simulink model "Temp_controlSysid"  (R2016b)
settings: Solver=FixedStepAuto  StartTime=0.0  StopTime=20000  RelTol=1e-3  EnableMultiTasking=on
undefined symbols (not defined in the file or in its folder): DiscIntNeverNeededParam
libraries: simulink x35, simulink_need_slupdate x5, EEE481Arduino x1
settings Model: ExtModeTrigDuration=2  Creator=EliteBook 8470p  LastModifiedBy=rsjoshi1
settings OptimizationCC: LifeSpan=1  MaxStackSize=64
settings DebuggingCC: SFUnexpectedBacktrackingDiag=warning  SFNoUnconditionalDefaultTransitionDiag=warning  SFExecutionAtInitializationDiag=none
settings HardwareCC: ProdBitPerPointer=32  ProdBitPerSizeT=32  ProdBitPerPtrDiffT=32  ProdLargestAtomicInteger=Long  ProdLargestAtomicFloat=Double  ProdWordSize=32  ProdHWDeviceType=ARM Compatible->ARM Cortex
settings RTWCC: SystemTargetFile=ert.tlc  HardwareBoard=Arduino Due  TLCOptions=-aInlineSetEventsForThisBaseRateFcn=TLC_FALSE -aSuppressMultiTaskScheduler=TLC_FALSE -aRateBasedStepFcn=1  TemplateMakefile=ert_default_tmf  Description=Embedded Coder  GenerateReport=on  Toolchain=Arduino ARM v1.6.7  BuildConfiguration=Faster Runs  IncludeHyperlinkInReport=on  LaunchReport=on  GenerateTraceInfo=on  GenerateTraceReport=on  GenerateTraceReportSl=on  GenerateTraceReportSf=on  GenerateTraceReportEml=on
settings CodeAppCC: ForceParamTrailComments=on  IgnoreCustomStorageClasses=off  OperatorAnnotations=on  SimulinkDataObjDesc=on  SFDataObjDesc=on  MATLABFcnDesc=on  InsertBlockDesc=on  MATLABSourceComments=on
settings ERTTargetCC: SupportContinuousTime=on  SupportVariableSizeSignals=on
settings ConfigComp: CovMetricSettings=dw  CovHtmlReporting=on  CovSaveCumulativeToWorkspaceVar=on  CovSaveSingleToWorkspaceVar=on  CovExternalEMLEnable=off

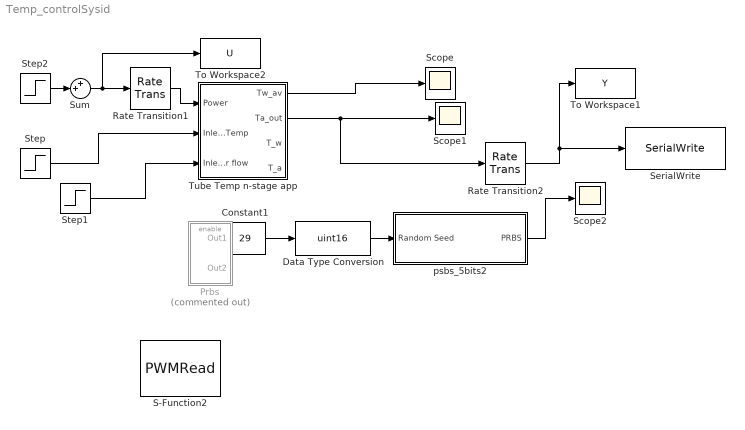
== system Temp_controlSysid ==
  Constant1 : Constant  Value=29  OutDataTypeStr=double  SampleTime=1
  Data Type Conversion : DataTypeConversion  OutDataTypeStr=uint16
  Prbs : Subsystem  Commented=on
  Rate Transition1 : RateTransition  OutPortSampleTimeOpt=Inherit  OutPortSampleTime=0.05
  Rate Transition2 : RateTransition  OutPortSampleTimeOpt=Inherit  OutPortSampleTime=0.05
  S-Function2 : S-Function  FunctionName=PWMRead  SFunctionModules=PWMRead_wrapper  SFunctionDeploymentMode=off  EnableBusSupport=off
  Scope : Scope
  Scope1 : Scope
  Scope2 : Scope
  SerialWrite : EEE481Arduino/SerialWrite  serialNum=2
  Step : Step  Time=10000  Before=25  After=25  SampleTime=0
  Step1 : Step  Time=5000  Before=1  SampleTime=0
  Step2 : Step  Time=100  After=0.49  SampleTime=1
  Sum : Sum  Inputs=++|
  To Workspace1 : ToWorkspace  VariableName=Y  SampleTime=1
  To Workspace2 : ToWorkspace  VariableName=U  SampleTime=1
  Tube Temp n-stage app : Subsystem  mask{L=0.5, n=10, ra=0.1, T_01=800, T_a01=25, T_amb=25}
      mask prompts: L "Tube Length"; n "Number of sections"; ra "Tube inner radius"; T_01 "Initial tube temp"; T_a01 "Initial air temp"; T_amb "Ambient Temp"
      mask init:
      | cp=1078;cpa=1134;rhoa=0.5;hs=5;ha=30;rhos=2500;k=2;
      | d=.01;vt=pi*L*((ra+d)*(ra+d)-ra*ra);m=vt*rhos;
      | As=2*pi*(ra+.1)*L;V=pi*ra*ra*L;Aa=2*pi*ra*L;
      | A_d=pi*((ra+d)*(ra+d)-ra*ra);A_rat=1;Li=L/n;
      | T_0=T_01*ones(n,1);T_a0=T_a01*ones(n,1);
  psbs_5bits2 : Subsystem  mask(PRBS with 8 shift registers){T=1, Tsw=200, Lz=12000, Lv=0.1, Nc=1}
      mask prompts: T "Sample Time (s)"; Tsw "Time to switch (s)"; Lz "Leading Zeros (s)"; Lv "Switching Levels"; Nc "Number of Cycles"
      mask help:
      | Creates a PRBS signal using 6 shift registers.
      |     *Time to switch (Tsw) must be an integer multiple of Sample Time (T).
      |     *Leading zeros specify how long the PRBS will be zero, in seconds, before the levels begin shifting.
      |     *Level is the amplitude of the desired PRBS signal. Both + and - levels are equal
      |     *Number of cycles determines the number of full cycles generated. Each cycle is (2^6-1)*Tsw seconds long
  wires:
  Step1/1 -> Tube Temp n-stage app/3(Inlet Air flow)
  Step/1 -> Tube Temp n-stage app/2(Inlet Air Temp)
  Tube Temp n-stage app/2(Ta_out) -> Rate Transition2/1, Scope1/1
  Tube Temp n-stage app/1(Tw_av) -> Scope/1
  psbs_5bits2/1(PRBS) -> Scope2/1
  Constant1/1 -> Data Type Conversion/1
  Data Type Conversion/1 -> psbs_5bits2/1(Random Seed)
  Step2/1 -> Sum/2
  Sum/1 -> To Workspace2/1, Rate Transition1/1
  Rate Transition1/1 -> Tube Temp n-stage app/1(Power)
  Rate Transition2/1 -> To Workspace1/1, SerialWrite/1

== system Temp_controlSysid/Prbs ==
  Enable : EnablePort
  Constant1 : Constant  Value=29  OutDataTypeStr=double  SampleTime=0.1
  Constant2 : Constant  Value=30  OutDataTypeStr=double  SampleTime=0.1
  Data Type Conversion : DataTypeConversion  OutDataTypeStr=uint16
  Data Type Conversion2 : DataTypeConversion  OutDataTypeStr=uint16
  Rate Transition1 : RateTransition  OutPortSampleTime=0.1
  Rate Transition2 : RateTransition  OutPortSampleTime=0.1
  psbs_5bits1 : Subsystem  mask(PRBS with 8 shift registers){T=0.1, Tsw=20, Lz=10, Lv=300, Nc=1}
      mask prompts: T "Sample Time (s)"; Tsw "Time to switch (s)"; Lz "Leading Zeros (s)"; Lv "Switching Levels"; Nc "Number of Cycles"
      mask help:
      | Creates a PRBS signal using 6 shift registers.
      |     *Time to switch (Tsw) must be an integer multiple of Sample Time (T).
      |     *Leading zeros specify how long the PRBS will be zero, in seconds, before the levels begin shifting.
      |     *Level is the amplitude of the desired PRBS signal. Both + and - levels are equal
      |     *Number of cycles determines the number of full cycles generated. Each cycle is (2^6-1)*Tsw seconds long
  psbs_5bits2 : Subsystem  mask(PRBS with 8 shift registers){T=0.1, Tsw=20, Lz=10, Lv=300, Nc=1}
      mask prompts: T "Sample Time (s)"; Tsw "Time to switch (s)"; Lz "Leading Zeros (s)"; Lv "Switching Levels"; Nc "Number of Cycles"
      mask help:
      | Creates a PRBS signal using 6 shift registers.
      |     *Time to switch (Tsw) must be an integer multiple of Sample Time (T).
      |     *Leading zeros specify how long the PRBS will be zero, in seconds, before the levels begin shifting.
      |     *Level is the amplitude of the desired PRBS signal. Both + and - levels are equal
      |     *Number of cycles determines the number of full cycles generated. Each cycle is (2^6-1)*Tsw seconds long
  psbs_7bits1 : Subsystem  Commented=on  mask(PRBS with 8 shift registers){T=0.1, Tsw=60, Lz=10, Lv=300, Nc=1}
      mask prompts: T "Sample Time (s)"; Tsw "Time to switch (s)"; Lz "Leading Zeros (s)"; Lv "Switching Levels"; Nc "Number of Cycles"
      mask help:
      | Creates a PRBS signal using 7 shift registers.
      |     *Time to switch (Tsw) must be an integer multiple of Sample Time (T).
      |     *Leading zeros specify how long the PRBS will be zero, in seconds, before the levels begin shifting.
      |     *Level is the amplitude of the desired PRBS signal. Both + and - levels are equal
      |     *Number of cycles determines the number of full cycles generated. Each cycle is (2^7-1)*Tsw seconds long
  psbs_8bits2 : Subsystem  Commented=on  mask(PRBS with 8 shift registers){T=0.1, Tsw=20, Lz=50, Lv=300, Nc=1}
      mask prompts: T "Sample Time (s)"; Tsw "Time to switch (s)"; Lz "Leading Zeros (s)"; Lv "Switching Levels"; Nc "Number of Cycles"
      mask help:
      | Creates a PRBS signal using 8 shift registers.
      |     *Time to switch (Tsw) must be an integer multiple of Sample Time (T).
      |     *Leading zeros specify how long the PRBS will be zero, in seconds, before the levels begin shifting.
      |     *Level is the amplitude of the desired PRBS signal. Both + and - levels are equal
      |     *Number of cycles determines the number of full cycles generated. Each cycle is (2^8-1)*Tsw seconds long
  Out1 : Outport
  Out2 : Outport  Port=2
  wires:
  Constant1/1 -> Data Type Conversion/1
  Data Type Conversion/1 -> Rate Transition1/1
  psbs_5bits2/1(PRBS) -> Out1/1
  Rate Transition1/1 -> psbs_5bits2/1(Random Seed)
  psbs_5bits1/1(PRBS) -> Out2/1
  Rate Transition2/1 -> psbs_5bits1/1(Random Seed)
  Constant2/1 -> Data Type Conversion2/1
  Data Type Conversion2/1 -> Rate Transition2/1

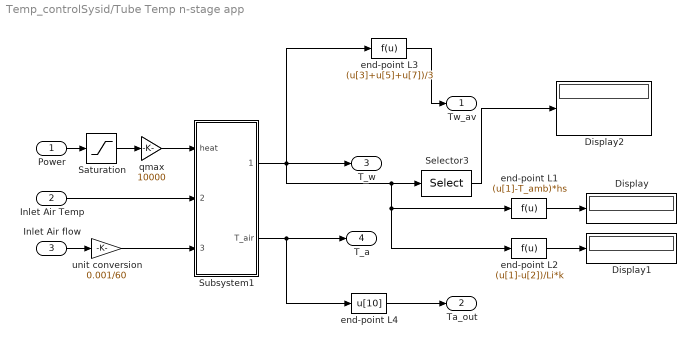
== system Temp_controlSysid/Tube Temp n-stage app ==
  Power : Inport
  Inlet Air Temp : Inport  Port=2
  Inlet Air flow : Inport  Port=3
  Display : Display
      settings: Format=short_e
  Display1 : Display
      settings: Format=short_e
  Display2 : Display
      settings: Format=short_e
  Saturation : Saturate  UpperLimit=1  LowerLimit=0
  Selector3 : Selector  InputPortWidth=n  IndexOptions=Index vector (dialog)  Indices=[1,2]  OutputSizes=1
  Subsystem1 : Subsystem
  end-point L1 : Fcn  Expr=(u[1]-T_amb)*hs
  end-point L2 : Fcn  Expr=(u[1]-u[2])/Li*k
  end-point L3 : Fcn  Expr=(u[3]+u[5]+u[7])/3
  end-point L4 : Fcn  Expr=u[10]
  qmax : Gain  Gain=10000  SaturateOnIntegerOverflow=on  OutDataTypeStr=Inherit: Same as input  ParamDataTypeStr=Inherit: Same as input
  unit conversion : Gain  Gain=0.001/60  SaturateOnIntegerOverflow=on  OutDataTypeStr=Inherit: Same as input  ParamDataTypeStr=Inherit: Same as input
  Tw_av : Outport
  Ta_out : Outport  Port=2
  T_w : Outport  Port=3
  T_a : Outport  Port=4
  wires:
  end-point L2/1 -> Display1/1
  end-point L1/1 -> Display/1
  Selector3/1 -> Display2/1
  Subsystem1/2(T_air) -> end-point L4/1, T_a/1
  Subsystem1/1(T_wall) -> end-point L3/1, end-point L2/1, end-point L1/1, Selector3/1, T_w/1
  unit conversion/1 -> Subsystem1/3(Air flow)
  Inlet Air flow/1 -> unit conversion/1
  Power/1 -> Saturation/1
  Saturation/1 -> qmax/1
  Inlet Air Temp/1 -> Subsystem1/2(T_a_inlet)
  qmax/1 -> Subsystem1/1(heat)
  end-point L3/1 -> Tw_av/1
  end-point L4/1 -> Ta_out/1

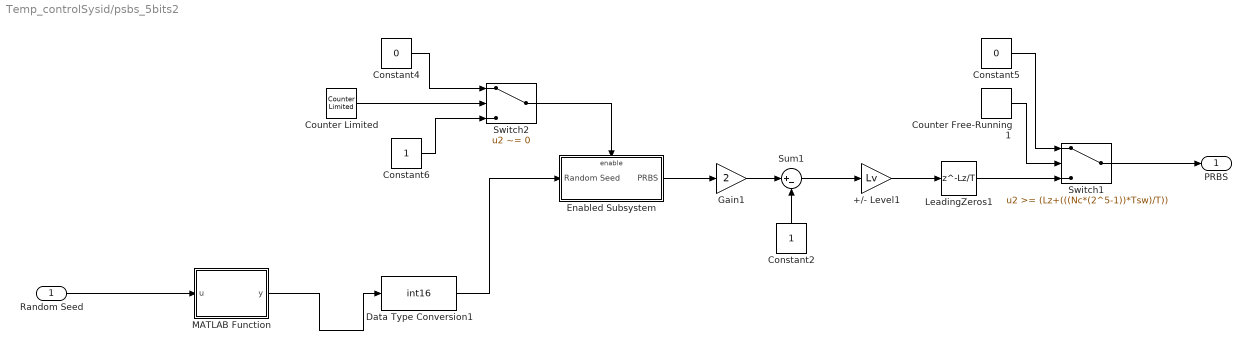
== system Temp_controlSysid/psbs_5bits2 ==
  Random Seed : Inport  OutDataTypeStr=uint16
  +/- Level1 : Gain  Gain=Lv  SampleTime=T
  Constant2 : Constant  SampleTime=T
  Constant4 : Constant  Value=0  SampleTime=T
  Constant5 : Constant  Value=0  SampleTime=T
  Constant6 : Constant  SampleTime=T
  Counter Free-Running1 : simulink/Sources/Counter Free-Running  NumBits=32  tsamp=T
  Counter Limited : simulink/Sources/Counter Limited  uplimit=Tsw/T-1  tsamp=T
  Data Type Conversion1 : DataTypeConversion  OutDataTypeStr=int16
  Enabled Subsystem : Subsystem  TreatAsAtomicUnit=on
  Gain1 : Gain  Gain=2  SampleTime=T
  LeadingZeros1 : Delay  DelayLength=Lz/T  InitialCondition=0  SampleTime=T
  MATLAB Function : MATLAB Function  TreatAsAtomicUnit=on
  Sum1 : Sum  Inputs=|+-  SampleTime=T
  Switch1 : Switch  Threshold=(Lz+(((Nc*(2^5-1))*Tsw)/T))  SampleTime=T
  Switch2 : Switch  Criteria=u2 ~= 0  Threshold=Tsw/T  SampleTime=T
  PRBS : Outport
  wires:
  Switch1/1 -> PRBS/1
  Random Seed/1 -> MATLAB Function/1(u)
  MATLAB Function/1(y) -> Data Type Conversion1/1
  LeadingZeros1/1 -> Switch1/3
  Constant5/1 -> Switch1/1
  +/- Level1/1 -> LeadingZeros1/1
  Counter Free-Running1/1 -> Switch1/2
  Constant2/1 -> Sum1/2
  Gain1/1 -> Sum1/1
  Sum1/1 -> +/- Level1/1
  Enabled Subsystem/1(PRBS) -> Gain1/1
  Data Type Conversion1/1 -> Enabled Subsystem/1(Random Seed)
  Constant6/1 -> Switch2/3
  Constant4/1 -> Switch2/1
  Switch2/1 -> Enabled Subsystem/Enable
  Counter Limited/1 -> Switch2/2

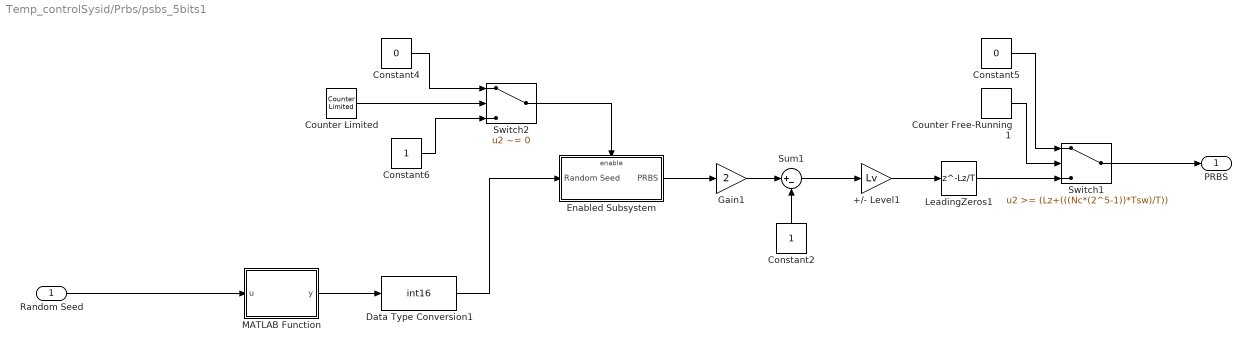
== system Temp_controlSysid/Prbs/psbs_5bits1 ==
  Random Seed : Inport  OutDataTypeStr=uint16
  +/- Level1 : Gain  Gain=Lv  SampleTime=T
  Constant2 : Constant  SampleTime=T
  Constant4 : Constant  Value=0  SampleTime=T
  Constant5 : Constant  Value=0  SampleTime=T
  Constant6 : Constant  SampleTime=T
  Counter Free-Running1 : simulink/Sources/Counter Free-Running  NumBits=32  tsamp=T
  Counter Limited : simulink/Sources/Counter Limited  uplimit=Tsw/T-1  tsamp=T
  Data Type Conversion1 : DataTypeConversion  OutDataTypeStr=int16
  Enabled Subsystem : Subsystem  TreatAsAtomicUnit=on
  Gain1 : Gain  Gain=2  SampleTime=T
  LeadingZeros1 : Delay  DelayLength=Lz/T  InitialCondition=0  SampleTime=T
  MATLAB Function : MATLAB Function  TreatAsAtomicUnit=on
  Sum1 : Sum  Inputs=|+-  SampleTime=T
  Switch1 : Switch  Threshold=(Lz+(((Nc*(2^5-1))*Tsw)/T))  SampleTime=T
  Switch2 : Switch  Criteria=u2 ~= 0  Threshold=Tsw/T  SampleTime=T
  PRBS : Outport
  wires:
  Counter Limited/1 -> Switch2/2
  Switch2/1 -> Enabled Subsystem/Enable
  Constant4/1 -> Switch2/1
  Constant6/1 -> Switch2/3
  Data Type Conversion1/1 -> Enabled Subsystem/1(Random Seed)
  Enabled Subsystem/1(PRBS) -> Gain1/1
  Sum1/1 -> +/- Level1/1
  Gain1/1 -> Sum1/1
  Constant2/1 -> Sum1/2
  Counter Free-Running1/1 -> Switch1/2
  +/- Level1/1 -> LeadingZeros1/1
  Constant5/1 -> Switch1/1
  LeadingZeros1/1 -> Switch1/3
  MATLAB Function/1(y) -> Data Type Conversion1/1
  Random Seed/1 -> MATLAB Function/1(u)
  Switch1/1 -> PRBS/1

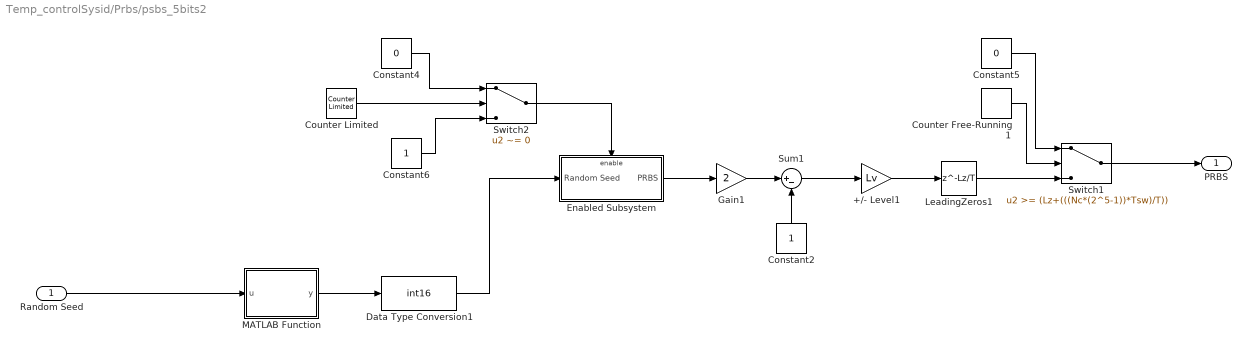
== system Temp_controlSysid/Prbs/psbs_5bits2 ==
  Random Seed : Inport  OutDataTypeStr=uint16
  +/- Level1 : Gain  Gain=Lv  SampleTime=T
  Constant2 : Constant  SampleTime=T
  Constant4 : Constant  Value=0  SampleTime=T
  Constant5 : Constant  Value=0  SampleTime=T
  Constant6 : Constant  SampleTime=T
  Counter Free-Running1 : simulink/Sources/Counter Free-Running  NumBits=32  tsamp=T
  Counter Limited : simulink/Sources/Counter Limited  uplimit=Tsw/T-1  tsamp=T
  Data Type Conversion1 : DataTypeConversion  OutDataTypeStr=int16
  Enabled Subsystem : Subsystem  TreatAsAtomicUnit=on
  Gain1 : Gain  Gain=2  SampleTime=T
  LeadingZeros1 : Delay  DelayLength=Lz/T  InitialCondition=0  SampleTime=T
  MATLAB Function : MATLAB Function  TreatAsAtomicUnit=on
  Sum1 : Sum  Inputs=|+-  SampleTime=T
  Switch1 : Switch  Threshold=(Lz+(((Nc*(2^5-1))*Tsw)/T))  SampleTime=T
  Switch2 : Switch  Criteria=u2 ~= 0  Threshold=Tsw/T  SampleTime=T
  PRBS : Outport
  wires:
  Switch1/1 -> PRBS/1
  Random Seed/1 -> MATLAB Function/1(u)
  MATLAB Function/1(y) -> Data Type Conversion1/1
  LeadingZeros1/1 -> Switch1/3
  Constant5/1 -> Switch1/1
  +/- Level1/1 -> LeadingZeros1/1
  Counter Free-Running1/1 -> Switch1/2
  Constant2/1 -> Sum1/2
  Gain1/1 -> Sum1/1
  Sum1/1 -> +/- Level1/1
  Enabled Subsystem/1(PRBS) -> Gain1/1
  Data Type Conversion1/1 -> Enabled Subsystem/1(Random Seed)
  Constant6/1 -> Switch2/3
  Constant4/1 -> Switch2/1
  Switch2/1 -> Enabled Subsystem/Enable
  Counter Limited/1 -> Switch2/2

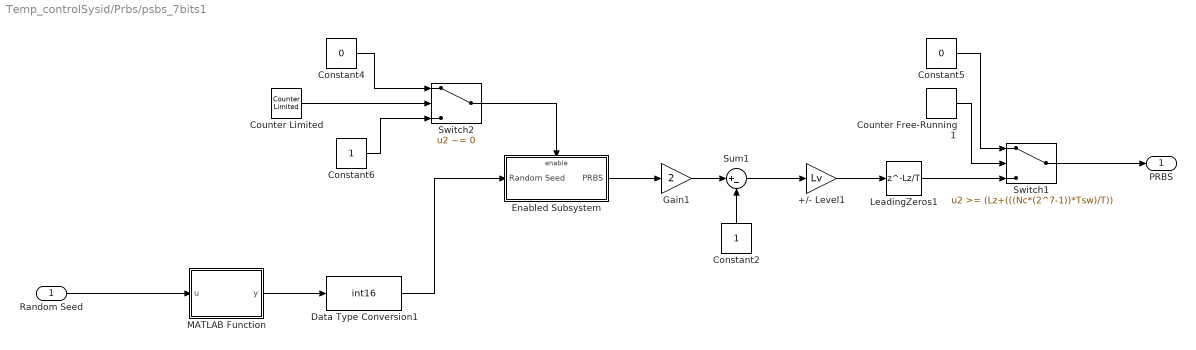
== system Temp_controlSysid/Prbs/psbs_7bits1 ==
  Random Seed : Inport  OutDataTypeStr=uint16
  +/- Level1 : Gain  Gain=Lv  SampleTime=T
  Constant2 : Constant  SampleTime=T
  Constant4 : Constant  Value=0  SampleTime=T
  Constant5 : Constant  Value=0  SampleTime=T
  Constant6 : Constant  SampleTime=T
  Counter Free-Running1 : simulink/Sources/Counter Free-Running  NumBits=32  tsamp=T
  Counter Limited : simulink/Sources/Counter Limited  uplimit=Tsw/T-1  tsamp=T
  Data Type Conversion1 : DataTypeConversion  OutDataTypeStr=int16
  Enabled Subsystem : Subsystem  TreatAsAtomicUnit=on
  Gain1 : Gain  Gain=2  SampleTime=T
  LeadingZeros1 : Delay  DelayLength=Lz/T  InitialCondition=0  SampleTime=T
  MATLAB Function : MATLAB Function  TreatAsAtomicUnit=on
  Sum1 : Sum  Inputs=|+-  SampleTime=T
  Switch1 : Switch  Threshold=(Lz+(((Nc*(2^7-1))*Tsw)/T))  SampleTime=T
  Switch2 : Switch  Criteria=u2 ~= 0  Threshold=Tsw/T  SampleTime=T
  PRBS : Outport
  wires:
  Switch1/1 -> PRBS/1
  Random Seed/1 -> MATLAB Function/1(u)
  MATLAB Function/1(y) -> Data Type Conversion1/1
  LeadingZeros1/1 -> Switch1/3
  Constant5/1 -> Switch1/1
  +/- Level1/1 -> LeadingZeros1/1
  Counter Free-Running1/1 -> Switch1/2
  Constant2/1 -> Sum1/2
  Gain1/1 -> Sum1/1
  Sum1/1 -> +/- Level1/1
  Enabled Subsystem/1(PRBS) -> Gain1/1
  Data Type Conversion1/1 -> Enabled Subsystem/1(Random Seed)
  Constant6/1 -> Switch2/3
  Constant4/1 -> Switch2/1
  Switch2/1 -> Enabled Subsystem/Enable
  Counter Limited/1 -> Switch2/2

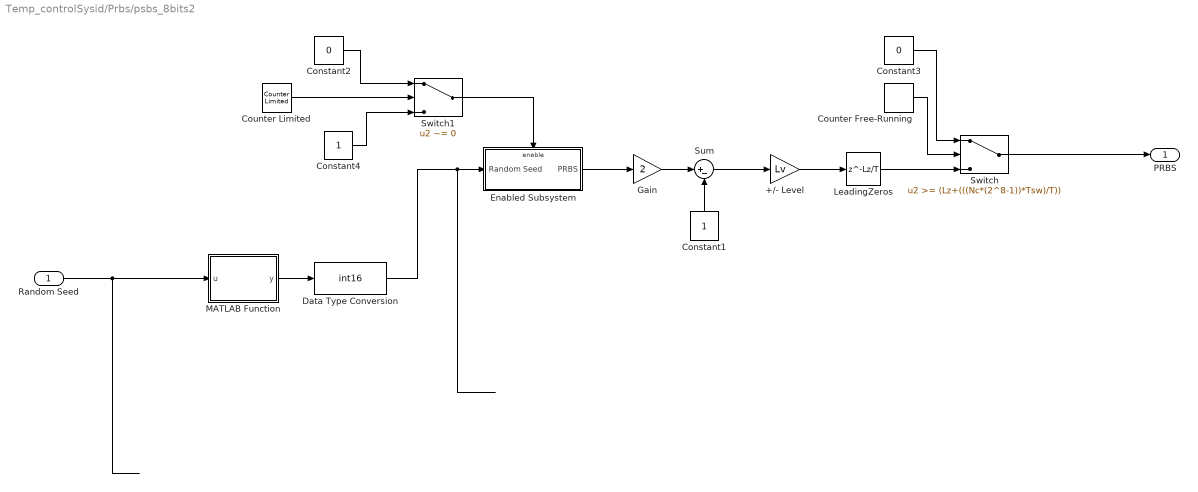
== system Temp_controlSysid/Prbs/psbs_8bits2 ==
  Random Seed : Inport  OutDataTypeStr=uint16  SampleTime=0.1
  +/- Level : Gain  Gain=Lv  SampleTime=T
  Constant1 : Constant  SampleTime=T
  Constant2 : Constant  Value=0  SampleTime=T
  Constant3 : Constant  Value=0  SampleTime=T
  Constant4 : Constant  SampleTime=T
  Counter Free-Running : simulink/Sources/Counter Free-Running  NumBits=32  tsamp=T
  Counter Limited : simulink/Sources/Counter Limited  uplimit=Tsw/T-1  tsamp=T
  Data Type Conversion : DataTypeConversion  OutDataTypeStr=int16
  Enabled Subsystem : Subsystem  TreatAsAtomicUnit=on
  Gain : Gain  Gain=2  SampleTime=T
  LeadingZeros : Delay  DelayLength=Lz/T  InitialCondition=0  SampleTime=T
  MATLAB Function : MATLAB Function  TreatAsAtomicUnit=on
  Sum : Sum  Inputs=|+-  SampleTime=T
  Switch : Switch  Threshold=(Lz+(((Nc*(2^8-1))*Tsw)/T))  SampleTime=T
  Switch1 : Switch  Criteria=u2 ~= 0  Threshold=Tsw/T  SampleTime=T
  PRBS : Outport
  wires:
  Switch/1 -> PRBS/1
  MATLAB Function/1(y) -> Data Type Conversion/1
  LeadingZeros/1 -> Switch/3
  Constant3/1 -> Switch/1
  +/- Level/1 -> LeadingZeros/1
  Counter Free-Running/1 -> Switch/2
  Constant1/1 -> Sum/2
  Gain/1 -> Sum/1
  Sum/1 -> +/- Level/1
  Enabled Subsystem/1(PRBS) -> Gain/1
  Data Type Conversion/1 -> Enabled Subsystem/1(Random Seed)
  Constant4/1 -> Switch1/3
  Constant2/1 -> Switch1/1
  Switch1/1 -> Enabled Subsystem/Enable
  Counter Limited/1 -> Switch1/2
  Random Seed/1 -> MATLAB Function/1(u)

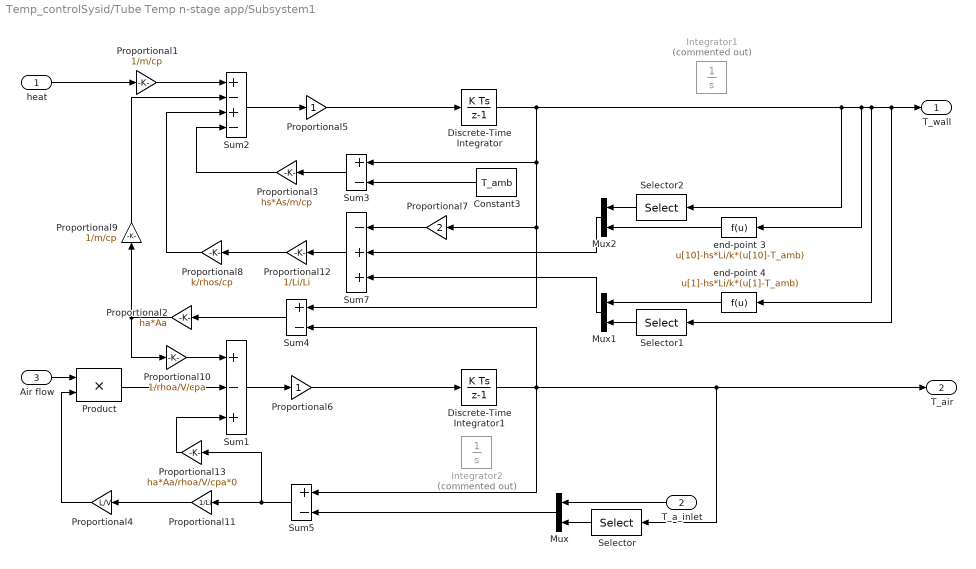
== system Temp_controlSysid/Tube Temp n-stage app/Subsystem1 ==
  heat : Inport
  T_a_inlet : Inport  Port=2
  Air flow : Inport  Port=3
  Constant3 : Constant  Value=T_amb
  Discrete-Time Integrator : DiscreteIntegrator  InitialCondition=T_0  InitialConditionSetting=State (most efficient)  SampleTime=0.05  ICPrevOutput=DiscIntNeverNeededParam  ICPrevScaledInput=DiscIntNeverNeededParam
  Discrete-Time Integrator1 : DiscreteIntegrator  InitialCondition=T_a0  InitialConditionSetting=State (most efficient)  SampleTime=0.05  ICPrevOutput=DiscIntNeverNeededParam  ICPrevScaledInput=DiscIntNeverNeededParam
  Integrator1 : Integrator  Commented=on  InitialCondition=T_0
  Integrator2 : Integrator  Commented=on  InitialCondition=T_a0
  Mux : Mux  Inputs=2
  Mux1 : Mux  Inputs=2
  Mux2 : Mux  Inputs=2
  Product : Product  SaturateOnIntegerOverflow=on  RndMeth=Zero  InputSameDT=on  OutDataTypeStr=Inherit: Same as first input
  Proportional1 : Gain  Gain=1/m/cp  SaturateOnIntegerOverflow=on  OutDataTypeStr=Inherit: Same as input  ParamDataTypeStr=Inherit: Same as input
  Proportional10 : Gain  Gain=1/rhoa/V/cpa  SaturateOnIntegerOverflow=on  OutDataTypeStr=Inherit: Same as input  ParamDataTypeStr=Inherit: Same as input
  Proportional11 : Gain  Gain=1/Li  SaturateOnIntegerOverflow=on  OutDataTypeStr=Inherit: Same as input  ParamDataTypeStr=Inherit: Same as input
  Proportional12 : Gain  Gain=1/Li/Li  SaturateOnIntegerOverflow=on  OutDataTypeStr=Inherit: Same as input  ParamDataTypeStr=Inherit: Same as input
  Proportional13 : Gain  Gain=ha*Aa/rhoa/V/cpa*0  SaturateOnIntegerOverflow=on  OutDataTypeStr=Inherit: Same as input  ParamDataTypeStr=Inherit: Same as input
  Proportional2 : Gain  Gain=ha*Aa  SaturateOnIntegerOverflow=on  OutDataTypeStr=Inherit: Same as input  ParamDataTypeStr=Inherit: Same as input
  Proportional3 : Gain  Gain=hs*As/m/cp  SaturateOnIntegerOverflow=on  OutDataTypeStr=Inherit: Same as input  ParamDataTypeStr=Inherit: Same as input
  Proportional4 : Gain  Gain=L/V  SaturateOnIntegerOverflow=on  OutDataTypeStr=Inherit: Same as input  ParamDataTypeStr=Inherit: Same as input
  Proportional5 : Gain  SaturateOnIntegerOverflow=on  OutDataTypeStr=Inherit: Same as input  ParamDataTypeStr=Inherit: Same as input
  Proportional6 : Gain  SaturateOnIntegerOverflow=on  OutDataTypeStr=Inherit: Same as input  ParamDataTypeStr=Inherit: Same as input
  Proportional7 : Gain  Gain=2  SaturateOnIntegerOverflow=on  OutDataTypeStr=Inherit: Same as input  ParamDataTypeStr=Inherit: Same as input
  Proportional8 : Gain  Gain=k/rhos/cp  SaturateOnIntegerOverflow=on  OutDataTypeStr=Inherit: Same as input  ParamDataTypeStr=Inherit: Same as input
  Proportional9 : Gain  Gain=1/m/cp  SaturateOnIntegerOverflow=on  OutDataTypeStr=Inherit: Same as input  ParamDataTypeStr=Inherit: Same as input
  Selector : Selector  InputPortWidth=n  IndexOptions=Index vector (dialog)  Indices=[1:n-1]  OutputSizes=1
  Selector1 : Selector  InputPortWidth=n  IndexOptions=Index vector (dialog)  Indices=[1:n-1]  OutputSizes=1
  Selector2 : Selector  InputPortWidth=n  IndexOptions=Index vector (dialog)  Indices=[2:n]  OutputSizes=1
  Sum1 : Sum  Inputs=+-+  SaturateOnIntegerOverflow=on  InputSameDT=on  OutDataTypeStr=Inherit: Same as first input
  Sum2 : Sum  Inputs=+-+-  SaturateOnIntegerOverflow=on  InputSameDT=on  OutDataTypeStr=Inherit: Same as first input
  Sum3 : Sum  Inputs=+-  SaturateOnIntegerOverflow=on  InputSameDT=on  OutDataTypeStr=Inherit: Same as first input
  Sum4 : Sum  Inputs=+-  SaturateOnIntegerOverflow=on  InputSameDT=on  OutDataTypeStr=Inherit: Same as first input
  Sum5 : Sum  Inputs=+-  SaturateOnIntegerOverflow=on  InputSameDT=on  OutDataTypeStr=Inherit: Same as first input
  Sum7 : Sum  Inputs=-++  SaturateOnIntegerOverflow=on  InputSameDT=on  OutDataTypeStr=Inherit: Same as first input
  end-point 3 : Fcn  Expr=u[10]-hs*Li/k*(u[10]-T_amb)
  end-point 4 : Fcn  Expr=u[1]-hs*Li/k*(u[1]-T_amb)
  T_wall : Outport
  T_air : Outport  Port=2
  wires:
  Proportional5/1 -> Discrete-Time Integrator/1
  Proportional3/1 -> Sum2/4
  Proportional13/1 -> Sum1/3
  end-point 3/1 -> Mux2/2
  end-point 4/1 -> Mux1/1
  Selector2/1 -> Mux2/1
  Selector1/1 -> Mux1/2
  Mux/1 -> Sum5/2
  Selector/1 -> Mux/2
  T_a_inlet/1 -> Mux/1
  Air flow/1 -> Product/1
  Product/1 -> Sum1/2
  Proportional4/1 -> Product/2
  Proportional12/1 -> Proportional8/1
  Proportional11/1 -> Proportional4/1
  Proportional10/1 -> Sum1/1
  Proportional9/1 -> Sum2/2
  Proportional1/1 -> Sum2/1
  Sum2/1 -> Proportional5/1
  Discrete-Time Integrator/1 -> end-point 3/1, end-point 4/1, Selector1/1, T_wall/1, Selector2/1, Sum3/1, Sum4/1, Proportional7/1
  Constant3/1 -> Sum3/2
  Sum3/1 -> Proportional3/1
  Sum4/1 -> Proportional2/1
  Proportional2/1 -> Proportional10/1, Proportional9/1
  Sum1/1 -> Proportional6/1
  Discrete-Time Integrator1/1 -> T_air/1, Selector/1, Sum4/2, Sum5/1
  Sum5/1 -> Proportional13/1, Proportional11/1
  heat/1 -> Proportional1/1
  Proportional6/1 -> Discrete-Time Integrator1/1
  Proportional7/1 -> Sum7/1
  Mux2/1 -> Sum7/2
  Mux1/1 -> Sum7/3
  Sum7/1 -> Proportional12/1
  Proportional8/1 -> Sum2/3

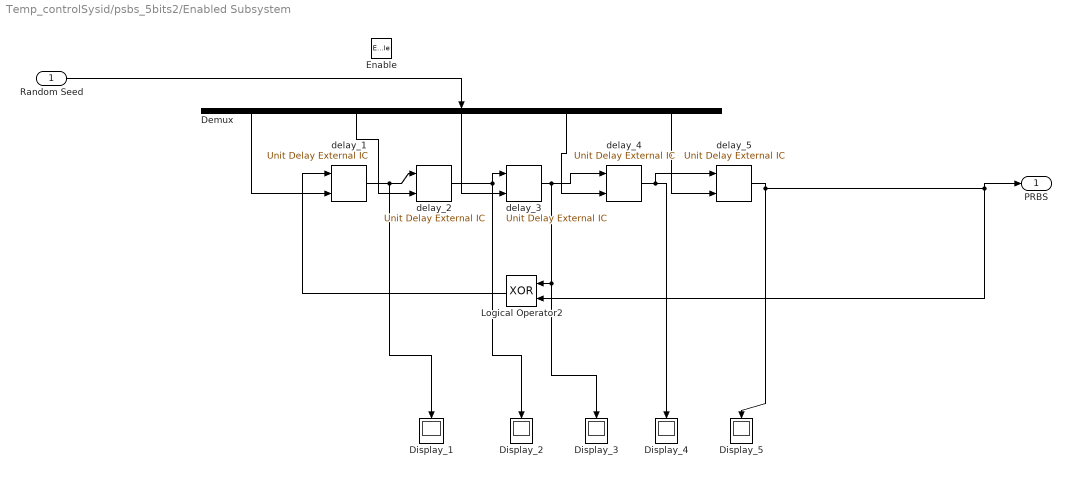
== system Temp_controlSysid/psbs_5bits2/Enabled Subsystem ==
  Random Seed : Inport  OutDataTypeStr=int16
  Enable : EnablePort
  Demux : Demux  Outputs=5
  Display_{1..5} (5 alike) : Display
  Logical Operator2 : Logic  Operator=XOR  AllPortsSameDT=off  OutDataTypeStr=fixdt(1,16)  SampleTime=T
  delay_{1..5} (5 alike) : simulink_need_slupdate/Unit Delay External IC  tsamp=T
  PRBS : Outport
  wires:
  delay_2/1 -> Display_2/1, delay_3/1
  delay_3/1 -> Display_3/1, Logical Operator2/1, delay_4/1
  delay_4/1 -> delay_5/1, Display_4/1
  delay_1/1 -> delay_2/1, Display_1/1
  Demux/5 -> delay_5/2
  Demux/4 -> delay_4/2
  Demux/3 -> delay_3/2
  Demux/2 -> delay_2/2
  Demux/1 -> delay_1/2
  Logical Operator2/1 -> delay_1/1
  delay_5/1 -> Display_5/1, PRBS/1, Logical Operator2/2
  Random Seed/1 -> Demux/1

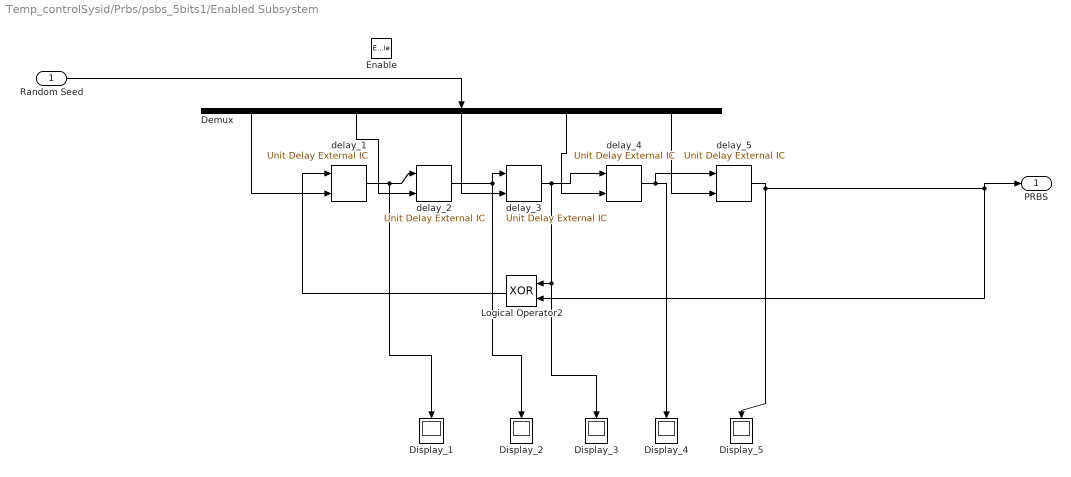
== system Temp_controlSysid/Prbs/psbs_5bits1/Enabled Subsystem ==
  Random Seed : Inport  OutDataTypeStr=int16
  Enable : EnablePort
  Demux : Demux  Outputs=5
  Display_{1..5} (5 alike) : Display
  Logical Operator2 : Logic  Operator=XOR  AllPortsSameDT=off  OutDataTypeStr=fixdt(1,16)  SampleTime=T
  delay_{1..5} (5 alike) : simulink/Additional Math & Discrete/Additional Discrete/Unit Delay External IC  tsamp=T
  PRBS : Outport
  wires:
  Random Seed/1 -> Demux/1
  delay_5/1 -> Logical Operator2/2, PRBS/1, Display_5/1
  Logical Operator2/1 -> delay_1/1
  Demux/1 -> delay_1/2
  Demux/2 -> delay_2/2
  Demux/3 -> delay_3/2
  Demux/4 -> delay_4/2
  Demux/5 -> delay_5/2
  delay_1/1 -> Display_1/1, delay_2/1
  delay_4/1 -> Display_4/1, delay_5/1
  delay_3/1 -> delay_4/1, Logical Operator2/1, Display_3/1
  delay_2/1 -> delay_3/1, Display_2/1

== system Temp_controlSysid/Prbs/psbs_5bits2/Enabled Subsystem ==
  Random Seed : Inport  OutDataTypeStr=int16
  Enable : EnablePort
  Demux : Demux  Outputs=5
  Display_{1..5} (5 alike) : Display
  Logical Operator2 : Logic  Operator=XOR  AllPortsSameDT=off  OutDataTypeStr=fixdt(1,16)  SampleTime=T
  delay_{1..5} (5 alike) : simulink/Additional Math & Discrete/Additional Discrete/Unit Delay External IC  tsamp=T
  PRBS : Outport
  wires:
  delay_2/1 -> Display_2/1, delay_3/1
  delay_3/1 -> Display_3/1, Logical Operator2/1, delay_4/1
  delay_4/1 -> delay_5/1, Display_4/1
  delay_1/1 -> delay_2/1, Display_1/1
  Demux/5 -> delay_5/2
  Demux/4 -> delay_4/2
  Demux/3 -> delay_3/2
  Demux/2 -> delay_2/2
  Demux/1 -> delay_1/2
  Logical Operator2/1 -> delay_1/1
  delay_5/1 -> Display_5/1, PRBS/1, Logical Operator2/2
  Random Seed/1 -> Demux/1

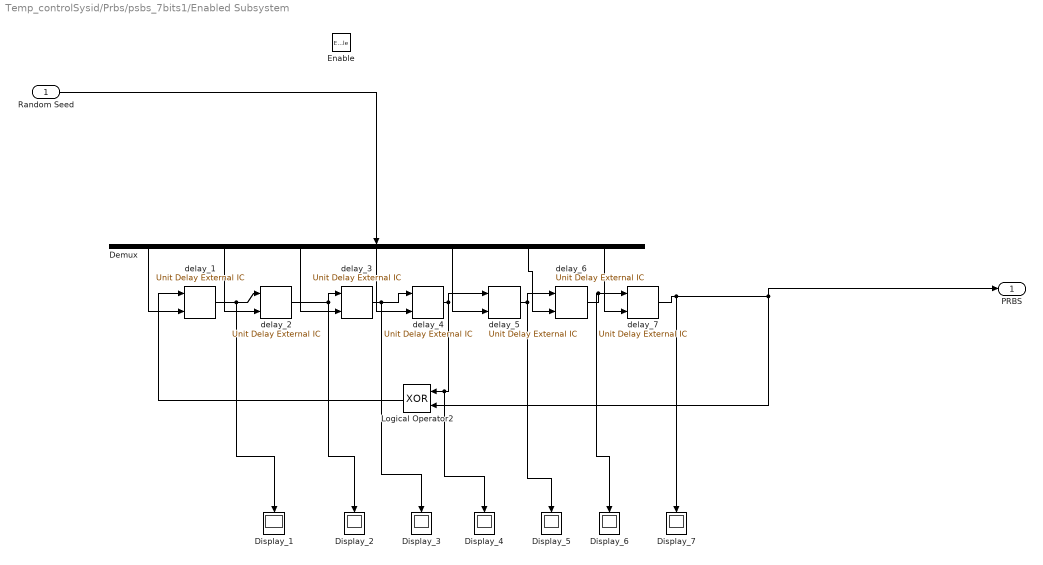
== system Temp_controlSysid/Prbs/psbs_7bits1/Enabled Subsystem ==
  Random Seed : Inport  OutDataTypeStr=int16
  Enable : EnablePort
  Demux : Demux  Outputs=7
  Display_{1..7} (7 alike) : Display
  Logical Operator2 : Logic  Operator=XOR  AllPortsSameDT=off  OutDataTypeStr=fixdt(1,16)  SampleTime=T
  delay_{1..7} (7 alike) : simulink/Additional Math & Discrete/Additional Discrete/Unit Delay External IC  tsamp=T
  PRBS : Outport
  wires:
  delay_7/1 -> Logical Operator2/2, PRBS/1, Display_7/1
  delay_5/1 -> Display_5/1, delay_6/1
  delay_6/1 -> Display_6/1, delay_7/1
  delay_2/1 -> Display_2/1, delay_3/1
  delay_3/1 -> Display_3/1, delay_4/1
  delay_4/1 -> Display_4/1, Logical Operator2/1, delay_5/1
  delay_1/1 -> delay_2/1, Display_1/1
  Demux/7 -> delay_7/2
  Demux/6 -> delay_6/2
  Demux/5 -> delay_5/2
  Demux/4 -> delay_4/2
  Demux/3 -> delay_3/2
  Demux/2 -> delay_2/2
  Demux/1 -> delay_1/2
  Random Seed/1 -> Demux/1
  Logical Operator2/1 -> delay_1/1

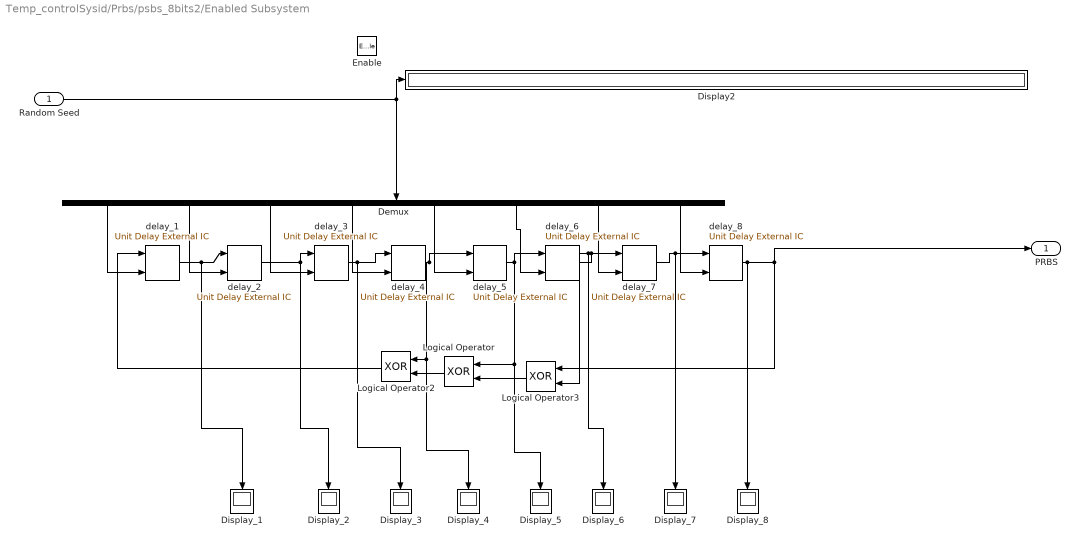
== system Temp_controlSysid/Prbs/psbs_8bits2/Enabled Subsystem ==
  Random Seed : Inport  OutDataTypeStr=int16
  Enable : EnablePort
  Demux : Demux  Outputs=8
  Display2 : Display
  Display_{1..8} (8 alike) : Display
  Logical Operator : Logic  Operator=XOR  AllPortsSameDT=off  OutDataTypeStr=fixdt(1,16)  SampleTime=T
  Logical Operator2 : Logic  Operator=XOR  AllPortsSameDT=off  OutDataTypeStr=fixdt(1,16)  SampleTime=T
  Logical Operator3 : Logic  Operator=XOR  AllPortsSameDT=off  OutDataTypeStr=fixdt(1,16)  SampleTime=T
  delay_{1..8} (8 alike) : simulink/Additional Math & Discrete/Additional Discrete/Unit Delay External IC  tsamp=T
  PRBS : Outport
  wires:
  delay_8/1 -> Display_8/1, PRBS/1, Logical Operator3/1
  Logical Operator2/1 -> delay_1/1
  Demux/1 -> delay_1/2
  Demux/2 -> delay_2/2
  Demux/3 -> delay_3/2
  Demux/4 -> delay_4/2
  Demux/5 -> delay_5/2
  Demux/6 -> delay_6/2
  Demux/7 -> delay_7/2
  Demux/8 -> delay_8/2
  Random Seed/1 -> Demux/1, Display2/1
  Logical Operator3/1 -> Logical Operator/2
  Logical Operator/1 -> Logical Operator2/2
  delay_7/1 -> delay_8/1, Display_7/1
  delay_1/1 -> Display_1/1, delay_2/1
  delay_4/1 -> delay_5/1, Logical Operator2/1, Display_4/1
  delay_3/1 -> delay_4/1, Display_3/1
  delay_2/1 -> delay_3/1, Display_2/1
  delay_6/1 -> delay_7/1, Display_6/1, Logical Operator3/2
  delay_5/1 -> delay_6/1, Logical Operator/1, Display_5/1

== matlab function Temp_controlSysid/Prbs/psbs_5bits2/MATLAB Function ==
  data: u input; y output
function y = fcn(u)
%#codegen
y = zeros(5,1);
% s = de2bi(u,16);
s = dec2bin(u,16);
y(1) = s(end-4)-48;
y(2) = s(end-3)-48;
y(3) = s(end-2)-48;
y(4) = s(end-1)-48;
y(5) = s(end)-48;

== matlab function Temp_controlSysid/psbs_5bits2/MATLAB Function ==
  data: u input; y output
function y = fcn(u)
%#codegen
y = zeros(5,1);
% s = de2bi(u,16);
s = dec2bin(u,16);
y(1) = s(end-4)-48;
y(2) = s(end-3)-48;
y(3) = s(end-2)-48;
y(4) = s(end-1)-48;
y(5) = s(end)-48;

== matlab function Temp_controlSysid/Prbs/psbs_5bits1/MATLAB Function ==
  data: u input; y output
function y = fcn(u)
%#codegen
y = zeros(5,1);
% s = de2bi(u,16);
s = dec2bin(u,16);
y(1) = s(end-4)-48;
y(2) = s(end-3)-48;
y(3) = s(end-2)-48;
y(4) = s(end-1)-48;
y(5) = s(end)-48;

== matlab function Temp_controlSysid/Prbs/psbs_7bits1/MATLAB Function ==
  data: u input; y output
function y = fcn(u)
%#codegen
y = zeros(7,1);
% s = de2bi(u,16);
s = dec2bin(u,16);
y(1) = s(end-6)-48;
y(2) = s(end-5)-48;
y(3) = s(end-4)-48;
y(4) = s(end-3)-48;
y(5) = s(end-2)-48;
y(6) = s(end-1)-48;
y(7) = s(end)-48;

== matlab function Temp_controlSysid/Prbs/psbs_8bits2/MATLAB Function ==
  data: u input; y output
function y = fcn(u)
%#codegen
y = zeros(8,1);
% s = de2bi(u,16);
s = dec2bin(u,16);
y(1) = s(end-7)-48;
y(2) = s(end-6)-48;
y(3) = s(end-5)-48;
y(4) = s(end-4)-48;
y(5) = s(end-3)-48;
y(6) = s(end-2)-48;
y(7) = s(end-1)-48;
y(8) = s(end)-48;
